simulink model "PB2M_001_003_RL"  (R2024a)
settings: Solver=FixedStepDiscrete  StartTime=0.0  StopTime=inf  FixedStep=[global_ST]  RelTol=1e-3
model workspace (MAT data in the model file):
  Var = 0
  imit_action_noise_variance = 0.2
values from neighbouring files (symbols this model uses):
  CGO2_cap = 5000    [SimControl_v3_rl.m]
  global_ST = 1    [SimControl_v3_rl.m]    (also in SimControl_v4.m)
  global_time = [0:1:8784]'    [SimControl_v3_rl.m]    (also in SimControl_v4.m)
undefined symbols (not defined in the file or in its folder): AEL, AMB, ATR, Bttry, CGO2, CHP, COMPR_MIX_E_spec, COMPR_SG_E_spec, DiscIntNeverNeededParam, DIST, DRY, forecast, GASF, Grd, MES, NumEpisodes, NumImitLearning, PV, th, vanilla, WT
libraries: simulink x1, slpidlib x1, rllib x1
(part 1 of 2)
settings Model: Creator=hogrebe  LastModifiedBy=salomon_p
settings SolverCC: AlgebraicLoopSolver=TrustRegion
settings DataIOCC: SaveState=on
settings OptimizationCC: BlockReduction=off
settings DebuggingCC: SignalInfNanChecking=error  UnconnectedInputMsg=warning  UnconnectedOutputMsg=warning  UnconnectedLineMsg=warning
settings ModelReferenceCC: EnableRefExpFcnMdlSchedulingChecks=on
settings RTWCC: GPUComputeCapability=3.5  DLArmComputeVersion=19.05

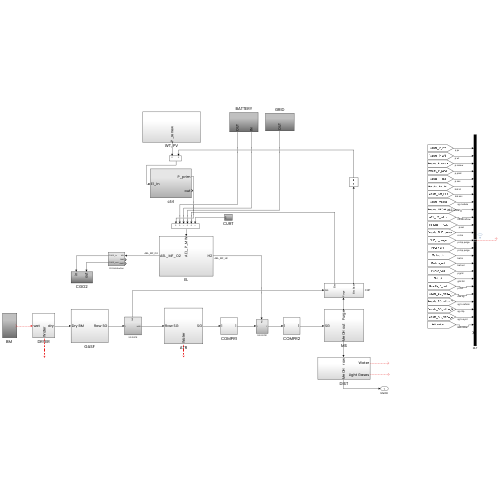
[thumbnail: Simulink's stored preview of the top-level diagram]
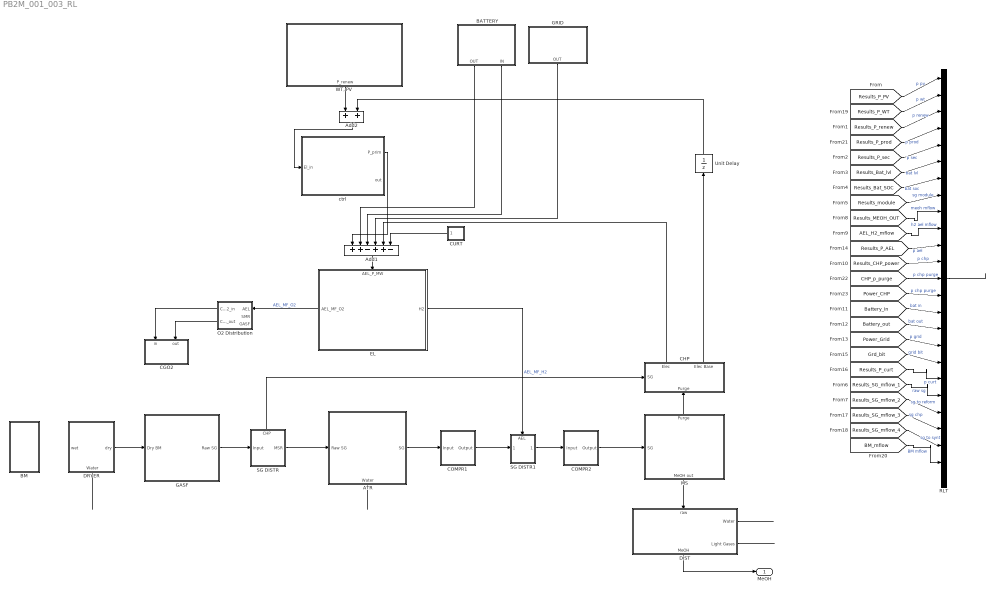
== system PB2M_001_003_RL ==
  ATR : Subsystem
      settings: PortSchema="{\"entries\":[{\"content\":{\"sides\":[{\"content\":{\"connectorIds\":[\"In1\"]},\"type\":\"ConnectorPlacement.EquallySpacedRectSide\",\"uuid\":\"d95d7370-a768-4e71-99c5-23d50f67aabe\"},{\"content\":{\"connectorIds\":[\"Out1\"],\"side\":\"RIGHT\"},\"type\":\"ConnectorPlacement.EquallySpacedRectSide\",\"uuid\":\"3437d418-ce7d-423d-8668-067a2caa5d39\"},{\"content\":{\"side\":\"TOP\"},\"type\":\"ConnectorPlacement.EquallySpacedRectSide\",\"uuid\":\"c8aa7c63-1393-4bbc-8660-d82006d9d42e\"},{\"content\":{\"connectorIds\":[\"Out2\"],\"side\":\"BOTTOM\"},\"type\":\"ConnectorPlacement.EquallySpacedRectSide\",\"uuid\":\"8d079498-92c7-4ac5-81b3-d100ec68b2bd\"}]},\"type\":\"ConnectorPlacement.EquallySpacedConnector\",\"uuid\":\"07712eec-a256-4c23-80e6-026550a38bce\"}],\"packageUris\":[\"http://schema.mathworks.com/mf0/Connector/R2020b\"],\"version\":\"1.0\"}"
  Add1 : Sum  Inputs=++-++-
  Add2 : Sum
  BATTERY : Subsystem
      settings: PortSchema="{\"entries\":[{\"content\":{\"sides\":[{\"content\":{},\"type\":\"ConnectorPlacement.EquallySpacedRectSide\",\"uuid\":\"b156ae25-26b3-4eee-ac7f-e302bdaac2ab\"},{\"content\":{\"side\":\"RIGHT\"},\"type\":\"ConnectorPlacement.EquallySpacedRectSide\",\"uuid\":\"f3a3b929-51c5-4419-b41e-ec6279a18565\"},{\"content\":{\"side\":\"TOP\"},\"type\":\"ConnectorPlacement.EquallySpacedRectSide\",\"uuid\":\"01f6443f-63f0-4718-804f-9bad3a04ddfb\"},{\"content\":{\"connectorIds\":[\"Out1\",\"Out2\"],\"side\":\"BOTTOM\"},\"type\":\"ConnectorPlacement.EquallySpacedRectSide\",\"uuid\":\"cbf48387-64e5-4e53-bde3-6e14dbb130f7\"}]},\"type\":\"ConnectorPlacement.EquallySpacedConnector\",\"uuid\":\"4aa34124-3e08-49a0-9db9-a8367ba9f9e9\"}],\"packageUris\":[\"http://schema.mathworks.com/mf0/Connector/R2020b\"],\"version\":\"1.0\"}"
  "BM " : Subsystem
  CGO2 : Subsystem
      settings: PortSchema="{\"entries\":[{\"content\":{\"sides\":[{\"content\":{},\"type\":\"ConnectorPlacement.EquallySpacedRectSide\",\"uuid\":\"5fd0e465-b758-40c5-99c0-bd502cf80220\"},{\"content\":{\"side\":\"RIGHT\"},\"type\":\"ConnectorPlacement.EquallySpacedRectSide\",\"uuid\":\"8c2bf71d-dd8a-4c38-9726-2100ecfb4157\"},{\"content\":{\"connectorIds\":[\"In1\",\"In2\"],\"side\":\"TOP\"},\"type\":\"ConnectorPlacement.EquallySpacedRectSide\",\"uuid\":\"9b00925e-eb9b-456e-968f-5d87047a8706\"}]},\"type\":\"ConnectorPlacement.EquallySpacedConnector\",\"uuid\":\"2f6cfec4-9fe2-41ff-9b0f-2d3a7383541d\"}],\"packageUris\":[\"http://schema.mathworks.com/mf0/Connector/R2020b\"],\"version\":\"1.0\"}"
  CHP : Subsystem
      settings: PortSchema="{\"entries\":[{\"content\":{\"sides\":[{\"content\":{\"connectorIds\":[\"In1\"]},\"type\":\"ConnectorPlacement.EquallySpacedRectSide\",\"uuid\":\"455e4cb2-b7ce-40b3-9267-45576cb92a35\"},{\"content\":{\"side\":\"RIGHT\"},\"type\":\"ConnectorPlacement.EquallySpacedRectSide\",\"uuid\":\"26266506-6e66-4bc0-bccd-a9e779dcae16\"},{\"content\":{\"connectorIds\":[\"Out1\",\"Out2\"],\"side\":\"TOP\"},\"type\":\"ConnectorPlacement.EquallySpacedRectSide\",\"uuid\":\"0bfe460e-97a8-4cdd-8918-1c56f22f3fbd\"},{\"content\":{\"connectorIds\":[\"In2\"],\"side\":\"BOTTOM\"},\"type\":\"ConnectorPlacement.EquallySpacedRectSide\",\"uuid\":\"d15a681e-1531-4d34-b913-d07bfab7e09a\"}]},\"type\":\"ConnectorPlacement.EquallySpacedConnector\",\"uuid\":\"864e4265-4fc9-4c94-8dd3-96a5c52575a2\"}],\"packageUris\":[\"http://schema.mathworks.com/mf0/Connector/R2020b\"],\"version\":\"1.0\"}"
  COMPR1 : Subsystem
  COMPR2 : Subsystem
  CURT : Subsystem
      settings: PortSchema="{\"entries\":[{\"content\":{\"sides\":[{\"content\":{\"connectorIds\":[\"Out1\"]},\"type\":\"ConnectorPlacement.EquallySpacedRectSide\",\"uuid\":\"455e4cb2-b7ce-40b3-9267-45576cb92a35\"},{\"content\":{\"side\":\"RIGHT\"},\"type\":\"ConnectorPlacement.EquallySpacedRectSide\",\"uuid\":\"26266506-6e66-4bc0-bccd-a9e779dcae16\"},{\"content\":{\"side\":\"TOP\"},\"type\":\"ConnectorPlacement.EquallySpacedRectSide\",\"uuid\":\"0bfe460e-97a8-4cdd-8918-1c56f22f3fbd\"}]},\"type\":\"ConnectorPlacement.EquallySpacedConnector\",\"uuid\":\"864e4265-4fc9-4c94-8dd3-96a5c52575a2\"}],\"packageUris\":[\"http://schema.mathworks.com/mf0/Connector/R2020b\"],\"version\":\"1.0\"}"
  DIST : Subsystem
      settings: PortSchema="{\"entries\":[{\"content\":{\"sides\":[{\"content\":{},\"type\":\"ConnectorPlacement.EquallySpacedRectSide\",\"uuid\":\"9bb20e76-c8c0-4ce3-bfa2-fd978c659bcc\"},{\"content\":{\"connectorIds\":[\"Out1\",\"Out2\"],\"side\":\"RIGHT\"},\"type\":\"ConnectorPlacement.EquallySpacedRectSide\",\"uuid\":\"12d31df4-77c9-4a5c-9a6c-fd7c89038c05\"},{\"content\":{\"connectorIds\":[\"In1\"],\"side\":\"TOP\"},\"type\":\"ConnectorPlacement.EquallySpacedRectSide\",\"uuid\":\"3a96496e-8d88-4b7f-91f0-6f8e8152b6d3\"},{\"content\":{\"connectorIds\":[\"Out3\"],\"side\":\"BOTTOM\"},\"type\":\"ConnectorPlacement.EquallySpacedRectSide\",\"uuid\":\"4bc833e2-fc0a-44a4-bcf0-3ebf0863e835\"}]},\"type\":\"ConnectorPlacement.EquallySpacedConnector\",\"uuid\":\"bb9c8f09-08c9-4a34-bdc9-5c844495fddc\"}],\"packageUris\":[\"http://schema.mathworks.com/mf0/Connector/R2020b\"],\"version\":\"1.0\"}"
  DRYER : Subsystem
      settings: PortSchema="{\"entries\":[{\"content\":{\"sides\":[{\"content\":{},\"type\":\"ConnectorPlacement.EquallySpacedRectSide\",\"uuid\":\"4ebfcccc-776f-4872-9d0b-9643b5960bad\"},{\"content\":{\"connectorIds\":[\"Out1\"],\"side\":\"RIGHT\"},\"type\":\"ConnectorPlacement.EquallySpacedRectSide\",\"uuid\":\"52af1a20-21ba-42da-ac0d-5cc3ed928415\"},{\"content\":{\"connectorIds\":[\"Out2\"],\"side\":\"TOP\"},\"type\":\"ConnectorPlacement.EquallySpacedRectSide\",\"uuid\":\"35b3f618-6f56-49d4-89a8-2314405479bc\"},{\"content\":{\"connectorIds\":[\"In1\"],\"side\":\"BOTTOM\"},\"type\":\"ConnectorPlacement.EquallySpacedRectSide\",\"uuid\":\"a7ad5d18-a31c-4405-a5bd-3fe59bb19813\"}]},\"type\":\"ConnectorPlacement.EquallySpacedConnector\",\"uuid\":\"90f717a7-269d-4abb-8032-a33661c35212\"}],\"packageUris\":[\"http://schema.mathworks.com/mf0/Connector/R2020b\"],\"version\":\"1.0\"}"
  EL : Subsystem
      settings: PortSchema="{\"entries\":[{\"content\":{\"sides\":[{\"content\":{\"connectorIds\":[\"Out2\"]},\"type\":\"ConnectorPlacement.EquallySpacedRectSide\",\"uuid\":\"e86b81d9-d45f-45ad-8c80-2ef5c9159145\"},{\"content\":{\"connectorIds\":[\"Out1\"],\"side\":\"RIGHT\"},\"type\":\"ConnectorPlacement.EquallySpacedRectSide\",\"uuid\":\"b091bd34-fe91-455d-8135-92fc1e1b5bd7\"},{\"content\":{\"connectorIds\":[\"In1\"],\"side\":\"TOP\"},\"type\":\"ConnectorPlacement.EquallySpacedRectSide\",\"uuid\":\"804c6318-ad33-4a07-b17e-e0d2fd6b4b2f\"}]},\"type\":\"ConnectorPlacement.EquallySpacedConnector\",\"uuid\":\"e581105a-7c66-468d-8489-1abddd5a4bb6\"}],\"packageUris\":[\"http://schema.mathworks.com/mf0/Connector/R2020b\"],\"version\":\"1.0\"}"
  GASF : Subsystem
  GRID : Subsystem
      settings: PortSchema="{\"entries\":[{\"content\":{\"sides\":[{\"content\":{},\"type\":\"ConnectorPlacement.EquallySpacedRectSide\",\"uuid\":\"13ddf689-c473-4fae-8488-05ba2c53be01\"},{\"content\":{\"side\":\"RIGHT\"},\"type\":\"ConnectorPlacement.EquallySpacedRectSide\",\"uuid\":\"3edd6540-09f8-47a0-8af0-925a1a207bbe\"},{\"content\":{\"side\":\"TOP\"},\"type\":\"ConnectorPlacement.EquallySpacedRectSide\",\"uuid\":\"e7e0af70-0c4e-4701-890f-2bc2f1b60263\"},{\"content\":{\"connectorIds\":[\"Out1\"],\"side\":\"BOTTOM\"},\"type\":\"ConnectorPlacement.EquallySpacedRectSide\",\"uuid\":\"aae9c7fc-ae1b-458f-888e-dcbddd5e368f\"}]},\"type\":\"ConnectorPlacement.EquallySpacedConnector\",\"uuid\":\"9fa59c12-9be8-49ba-a862-8cdac5f592f4\"}],\"packageUris\":[\"http://schema.mathworks.com/mf0/Connector/R2020b\"],\"version\":\"1.0\"}"
  MS : Subsystem
      settings: PortSchema="{\"entries\":[{\"content\":{\"sides\":[{\"content\":{\"connectorIds\":[\"In1\"]},\"type\":\"ConnectorPlacement.EquallySpacedRectSide\",\"uuid\":\"7c68cb95-e770-413e-a40e-672fd8604812\"},{\"content\":{\"side\":\"RIGHT\"},\"type\":\"ConnectorPlacement.EquallySpacedRectSide\",\"uuid\":\"6240a65a-2dbc-4a6e-817e-2ab31946396e\"},{\"content\":{\"connectorIds\":[\"Out2\"],\"side\":\"TOP\"},\"type\":\"ConnectorPlacement.EquallySpacedRectSide\",\"uuid\":\"1a1b519e-0693-45b9-a906-950b0dca57a1\"},{\"content\":{\"connectorIds\":[\"Out1\"],\"side\":\"BOTTOM\"},\"type\":\"ConnectorPlacement.EquallySpacedRectSide\",\"uuid\":\"e87dd805-e630-4a2f-8388-2c51cd14fe9e\"}]},\"type\":\"ConnectorPlacement.EquallySpacedConnector\",\"uuid\":\"e16e5d91-de04-48fc-b44b-fdb042a92f84\"}],\"packageUris\":[\"http://schema.mathworks.com/mf0/Connector/R2020b\"],\"version\":\"1.0\"}"
  O2 Distribution : Subsystem
      settings: PortSchema="{\"entries\":[{\"content\":{\"sides\":[{\"content\":{\"connectorIds\":[\"Out3\",\"Out4\"]},\"type\":\"ConnectorPlacement.EquallySpacedRectSide\",\"uuid\":\"30156f9c-db5e-4257-aeed-83f2c1c2e5bf\"},{\"content\":{\"connectorIds\":[\"In1\",\"Out1\",\"Out2\"],\"side\":\"RIGHT\"},\"type\":\"ConnectorPlacement.EquallySpacedRectSide\",\"uuid\":\"c3a4c4df-5b27-475f-87a9-b45da9a3b436\"},{\"content\":{\"side\":\"TOP\"},\"type\":\"ConnectorPlacement.EquallySpacedRectSide\",\"uuid\":\"5997053d-e240-46ef-b6d7-4f9a3a1c0d15\"}]},\"type\":\"ConnectorPlacement.EquallySpacedConnector\",\"uuid\":\"10d495fb-251b-444d-bd0a-f6bbcb16daf1\"}],\"packageUris\":[\"http://schema.mathworks.com/mf0/Connector/R2020b\"],\"version\":\"1.0\"}"
  RLT : BusCreator  Inputs=25
  SG DISTR : Subsystem
      settings: PortSchema="{\"entries\":[{\"content\":{\"sides\":[{\"content\":{},\"type\":\"ConnectorPlacement.EquallySpacedRectSide\",\"uuid\":\"e86b81d9-d45f-45ad-8c80-2ef5c9159145\"},{\"content\":{\"connectorIds\":[\"Out1\"],\"side\":\"RIGHT\"},\"type\":\"ConnectorPlacement.EquallySpacedRectSide\",\"uuid\":\"b091bd34-fe91-455d-8135-92fc1e1b5bd7\"},{\"content\":{\"connectorIds\":[\"In1\"],\"side\":\"TOP\"},\"type\":\"ConnectorPlacement.EquallySpacedRectSide\",\"uuid\":\"804c6318-ad33-4a07-b17e-e0d2fd6b4b2f\"},{\"content\":{\"connectorIds\":[\"Out2\"],\"side\":\"BOTTOM\"},\"type\":\"ConnectorPlacement.EquallySpacedRectSide\",\"uuid\":\"fb2b571c-70ad-41c0-9018-552f5e98e285\"}]},\"type\":\"ConnectorPlacement.EquallySpacedConnector\",\"uuid\":\"e581105a-7c66-468d-8489-1abddd5a4bb6\"}],\"packageUris\":[\"http://schema.mathworks.com/mf0/Connector/R2020b\"],\"version\":\"1.0\"}"
  SG DISTR1 : Subsystem
      settings: PortSchema="{\"entries\":[{\"content\":{\"sides\":[{\"content\":{},\"type\":\"ConnectorPlacement.EquallySpacedRectSide\",\"uuid\":\"e9c91cab-8c69-4152-b789-7325d2e32e4b\"},{\"content\":{\"connectorIds\":[\"In2\"],\"side\":\"RIGHT\"},\"type\":\"ConnectorPlacement.EquallySpacedRectSide\",\"uuid\":\"b801369b-5c93-4438-bd90-0992b326086c\"},{\"content\":{\"connectorIds\":[\"In1\"],\"side\":\"TOP\"},\"type\":\"ConnectorPlacement.EquallySpacedRectSide\",\"uuid\":\"e103e961-9a42-4e45-906c-e9068e5e276c\"},{\"content\":{\"connectorIds\":[\"Out1\"],\"side\":\"BOTTOM\"},\"type\":\"ConnectorPlacement.EquallySpacedRectSide\",\"uuid\":\"0e96afff-5922-401c-b36e-06eb0842909a\"}]},\"type\":\"ConnectorPlacement.EquallySpacedConnector\",\"uuid\":\"2ea93f77-6b27-4245-9c93-a72fb1fe7fa6\"}],\"packageUris\":[\"http://schema.mathworks.com/mf0/Connector/R2020b\"],\"version\":\"1.0\"}"
  Unit Delay : UnitDelay  SampleTime=-1  HasFrameUpgradeWarning=on
  "WT, PV" : Subsystem
      settings: PortSchema="{\"entries\":[{\"content\":{\"sides\":[{\"content\":{},\"type\":\"ConnectorPlacement.EquallySpacedRectSide\",\"uuid\":\"8a2d1ae0-dccb-4b14-8547-5eeedb1731af\"},{\"content\":{\"side\":\"RIGHT\"},\"type\":\"ConnectorPlacement.EquallySpacedRectSide\",\"uuid\":\"3fb157a2-f839-4f36-8a45-db822d022818\"},{\"content\":{\"side\":\"TOP\"},\"type\":\"ConnectorPlacement.EquallySpacedRectSide\",\"uuid\":\"528eda02-61b1-46fc-814d-d4347d4497c7\"},{\"content\":{\"connectorIds\":[\"Out1\"],\"side\":\"BOTTOM\"},\"type\":\"ConnectorPlacement.EquallySpacedRectSide\",\"uuid\":\"9515b46c-adb3-49ca-b783-afbfd8bcb61a\"}]},\"type\":\"ConnectorPlacement.EquallySpacedConnector\",\"uuid\":\"11973188-1db2-4f1c-be62-25a3f427210a\"}],\"packageUris\":[\"http://schema.mathworks.com/mf0/Connector/R2020b\"],\"version\":\"1.0\"}"
  ctrl : Subsystem
  MeOH : Outport
  wires:
  EL/2(AEL_MF_O2) -> O2 Distribution/1(AEL)  "AEL_MF_O2"
  O2 Distribution/4(CGO2_out) -> CGO2/2(out)
  O2 Distribution/3(CGO2_in) -> CGO2/1(in)
  SG DISTR/2(MSR) -> ATR/1(Raw SG)
  DRYER/2(dry) -> GASF/1(Dry BM)
  GASF/1(Raw SG) -> SG DISTR/1(Input)
  EL/1(H2) -> SG DISTR1/2(AEL)  "AEL_MF_H2"
  ATR/1(SG) -> COMPR1/1(Input)
  SG DISTR1/1(Output) -> COMPR2/1(Input)
  SG DISTR/1(CHP) -> CHP/1(SG)
  ? -> DRYER/1(wet)
  COMPR2/1(Output) -> MS/1(SG)
  ctrl/1(P_prim) -> Add1/1
  Add1/1 -> EL/1(AEL_P_MW)
  CHP/1(Elec) -> Add1/5
  BATTERY/1(OUT) -> Add1/2
  BATTERY/2(IN) -> Add1/3
  GRID/1(OUT) -> Add1/4
  CURT/1(Output) -> Add1/6
  COMPR1/1(Output) -> SG DISTR1/1(Input1)
  RLT/1 -> ?
  [Results_SG_mflow_4] -> RLT/23  "sg to synt"
  [Results_SG_mflow_2] -> RLT/21  "sg to reform"
  [Results_P_curt] -> RLT/19  "p curt"
  [Results_P_PV] -> RLT/1  "p pv"
  [Grd_bit] -> RLT/18  "grid bit"
  [Results_P_renew] -> RLT/3  "p renew"
  [Power_Grid] -> RLT/17  "p grid"
  [Results_CHP_power] -> RLT/12  "p chp"
  [Battery_out] -> RLT/16  "bat out"
  [Results_module] -> RLT/8  "sg module"
  [Battery_in] -> RLT/15  "bat in"
  [Results_P_AEL] -> RLT/11  "p ael"
  [AEL_H2_mflow] -> RLT/10  "h2 ael mflow"
  [Results_Bat_SOC] -> RLT/7  "bat soc"
  [Results_Bat_lvl] -> RLT/6  "bat lvl"
  [Results_MEOH_OUT] -> RLT/9  "meoh mflow"
  [Results_SG_mflow_1] -> RLT/20  "raw sg"
  [Results_P_sec] -> RLT/5  "p sec"
  [Results_SG_mflow_3] -> RLT/22  "sg chp"
  MS/2(Purge) -> CHP/2(Purge)
  Add2/1 -> ctrl/1(El_in)
  "WT, PV"/1(P_renew) -> Add2/1
  CHP/2(Elec Base) -> Unit Delay/1
  DRYER/1(Water) -> ?
  ATR/2(Water) -> ?
  MS/1(MeOH out) -> DIST/1(raw)
  DIST/3(MeOH) -> MeOH/1
  DIST/1(Water) -> ?
  DIST/2(Light Gases) -> ?
  [BM_mflow] -> RLT/24  "BM mflow"
  [Results_P_prod] -> RLT/4  "p prod"
  [CHP_p_purge] -> RLT/13  "p chp purge"
  [Power_CHP] -> RLT/14  "p chp purge"
  [Results_P_WT] -> RLT/2  "p wt"
  Unit Delay/1 -> Add2/2

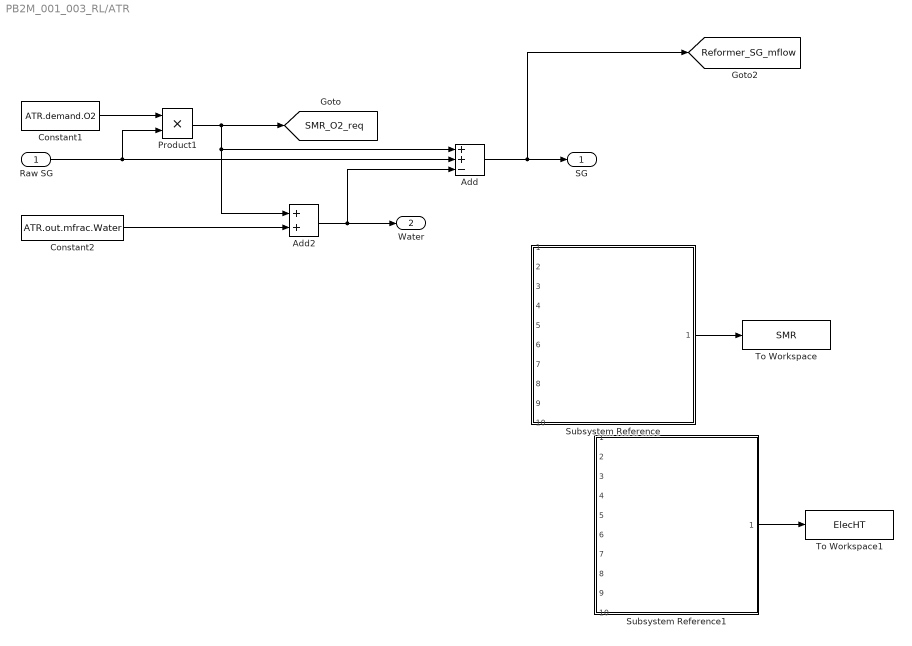
== system PB2M_001_003_RL/ATR ==
  Raw SG : Inport
  Add : Sum  Inputs=++-
  Add2 : Sum
  Constant1 : Constant  Value=ATR.demand.O2
  Constant2 : Constant  Value=ATR.out.mfrac.Water
  Product1 : Product
  Subsystem Reference : Subsystem  ReferencedSubsystem=Output_generation
  Subsystem Reference1 : Subsystem  ReferencedSubsystem=Output_generation
  To Workspace : ToWorkspace  VariableName=SMR  SampleTime=-1
  To Workspace1 : ToWorkspace  VariableName=ElecHT  SampleTime=-1
  SG : Outport
  Water : Outport  Port=2
  tag scope: Reformer_SG_mflow=global, SMR_O2_req=global
  wires:
  Subsystem Reference/1 -> To Workspace/1
  Constant1/1 -> Product1/1
  Product1/1 -> Add/1, Add2/1, [SMR_O2_req]
  Raw SG/1 -> Add/2, Product1/2
  Constant2/1 -> Add2/2
  Add2/1 -> Add/3, Water/1
  Add/1 -> [Reformer_SG_mflow], SG/1
  Subsystem Reference1/1 -> To Workspace1/1

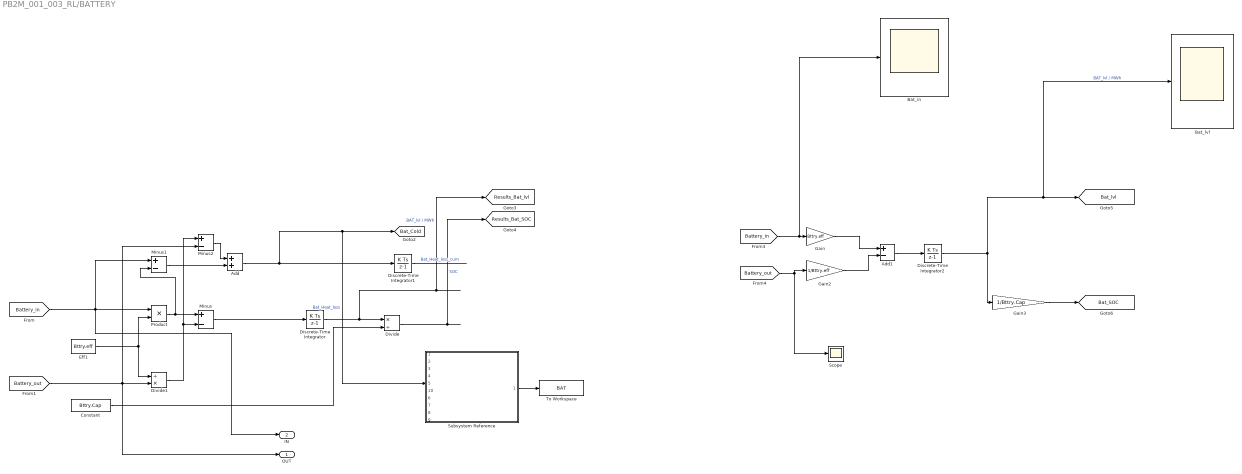
== system PB2M_001_003_RL/BATTERY ==
  Add : Sum
  Add1 : Sum  Inputs=+-
  Bat_in : Scope
  Bat_lvl : Scope
  Constant : Constant  Value=Bttry.Cap
  Discrete-Time Integrator : DiscreteIntegrator  SampleTime=-1  ICPrevOutput=DiscIntNeverNeededParam  ICPrevScaledInput=DiscIntNeverNeededParam
  Discrete-Time Integrator1 : DiscreteIntegrator  SampleTime=-1  ICPrevOutput=DiscIntNeverNeededParam  ICPrevScaledInput=DiscIntNeverNeededParam
  Discrete-Time Integrator2 : DiscreteIntegrator  InitialCondition=Bttry.min  SampleTime=-1  LimitOutput=on  UpperSaturationLimit=Bttry.Cap  LowerSaturationLimit=Bttry.min  ICPrevOutput=DiscIntNeverNeededParam  ICPrevScaledInput=DiscIntNeverNeededParam
  Divide : Product  Inputs=*/
  Divide1 : Product  Inputs=/*
  Eff1 : Constant  Value=Bttry.eff
  Gain : Gain  Gain=Bttry.eff
  Gain2 : Gain  Gain=1/Bttry.eff
  Gain3 : Gain  Gain=1/Bttry.Cap
  Minus : Sum  Inputs=+-
  Minus1 : Sum  Inputs=+-
  Minus2 : Sum  Inputs=+-
  Product : Product
  Scope : Scope
  Subsystem Reference : Subsystem  ReferencedSubsystem=Output_generation
      settings: PortSchema="{\"entries\":[{\"content\":{\"sides\":[{\"content\":{\"connectorIds\":[\"In1\",\"In2\",\"In3\",\"In4\",\"In5\",\"In10\",\"In6\",\"In7\",\"In8\",\"In9\"]},\"type\":\"ConnectorPlacement.EquallySpacedRectSide\",\"uuid\":\"21c211f6-d300-429e-920b-eada30affdb6\"},{\"content\":{\"connectorIds\":[\"Out1\"],\"side\":\"RIGHT\"},\"type\":\"ConnectorPlacement.EquallySpacedRectSide\",\"uuid\":\"b1fcdfee-52f7-4682-8799-22b33d08abbf\"},{\"content\":{\"side\":\"TOP\"},\"type\":\"ConnectorPlacement.EquallySpacedRectSide\",\"uuid\":\"5cecd853-e592-48b7-a1a6-516483ee8138\"}]},\"type\":\"ConnectorPlacement.EquallySpacedConnector\",\"uuid\":\"0d6337ce-2718-4de2-80e8-a88f22d313ea\"}],\"packageUris\":[\"http://schema.mathworks.com/mf0/Connector/R2020b\"],\"version\":\"1.0\"}"
  To Workspace : ToWorkspace  VariableName=BAT  SampleTime=-1
  OUT : Outport
  IN : Outport  Port=2
  tag scope: Bat_Cold=global, Bat_SOC=global, Bat_lvl=global, Results_Bat_SOC=global, Results_Bat_lvl=global
  wires:
  Constant/1 -> Divide/2
  Divide/1 -> [Results_Bat_SOC]  "SOC"
  Product/1 -> Minus1/2, Minus/1
  Divide1/1 -> Minus2/1, Minus/2
  Eff1/1 -> Divide1/1, Product/2
  Discrete-Time Integrator/1 -> [Results_Bat_lvl], Divide/1  "BAT_lvl / MWh"
  Subsystem Reference/1 -> To Workspace/1
  Minus1/1 -> Add/2
  Minus2/1 -> Add/1
  Add/1 -> [Bat_Cold], Subsystem Reference/5, Discrete-Time Integrator1/1  "Bat_Heat_loss"
  Discrete-Time Integrator1/1 -> ?  "Bat_Heat_loss_cum"
  [Battery_out] -> Divide1/2, OUT/1, Minus2/2
  [Battery_in] -> IN/1, Minus1/1, Product/1
  Minus/1 -> Discrete-Time Integrator/1
  [Battery_in] -> Bat_in/1, Gain/1
  [Battery_out] -> Scope/1, Gain2/1
  Gain2/1 -> Add1/2
  Add1/1 -> Discrete-Time Integrator2/1
  Gain/1 -> Add1/1
  Discrete-Time Integrator2/1 -> Bat_lvl/1, [Bat_lvl], Gain3/1  "BAT_lvl / MWh"
  Gain3/1 -> [Bat_SOC]

== system PB2M_001_003_RL/BM  ==
  IC : InitialCondition
  MATLAB Function : MATLAB Function  TreatAsAtomicUnit=on
  Unit Delay : UnitDelay  SampleTime=-1  HasFrameUpgradeWarning=on
  Unit Delay1 : UnitDelay  SampleTime=-1  HasFrameUpgradeWarning=on
  tag scope: Results_module=global
  wires:
  [AEL_H2_mflow] -> Unit Delay/1
  [Reformer_SG_mflow] -> Unit Delay1/1
  MATLAB Function/1(module) -> IC/1
  IC/1 -> [Results_module]
  Unit Delay/1 -> MATLAB Function/1(mflow_H2)
  Unit Delay1/1 -> MATLAB Function/2(mflow_SG)

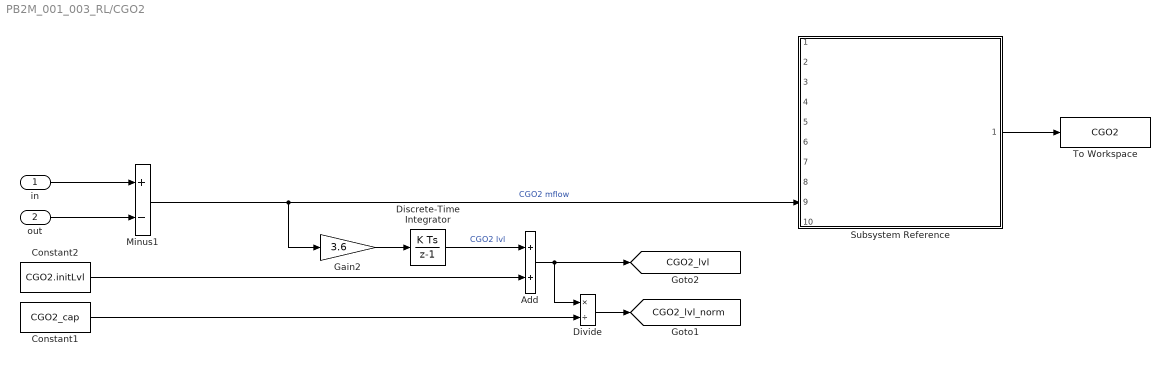
== system PB2M_001_003_RL/CGO2 ==
  in : Inport
  out : Inport  Port=2
  Add : Sum
  Constant1 : Constant  Value=CGO2_cap
  Constant2 : Constant  Value=CGO2.initLvl
  Discrete-Time Integrator : DiscreteIntegrator  SampleTime=-1  ICPrevOutput=DiscIntNeverNeededParam  ICPrevScaledInput=DiscIntNeverNeededParam
  Divide : Product  Inputs=*/
  Gain2 : Gain  Gain=3.6
  Minus1 : Sum  Inputs=+-
  Subsystem Reference : Subsystem  ReferencedSubsystem=Output_generation
  To Workspace : ToWorkspace  VariableName=CGO2  SampleTime=-1
  tag scope: CGO2_lvl=global, CGO2_lvl_norm=global
  wires:
  in/1 -> Minus1/1
  out/1 -> Minus1/2
  Minus1/1 -> Gain2/1, Subsystem Reference/9  "CGO2 mflow"
  Subsystem Reference/1 -> To Workspace/1
  Gain2/1 -> Discrete-Time Integrator/1
  Discrete-Time Integrator/1 -> Add/1  "CGO2 lvl"
  Constant2/1 -> Add/2
  Add/1 -> Divide/1, [CGO2_lvl]
  Constant1/1 -> Divide/2
  Divide/1 -> [CGO2_lvl_norm]

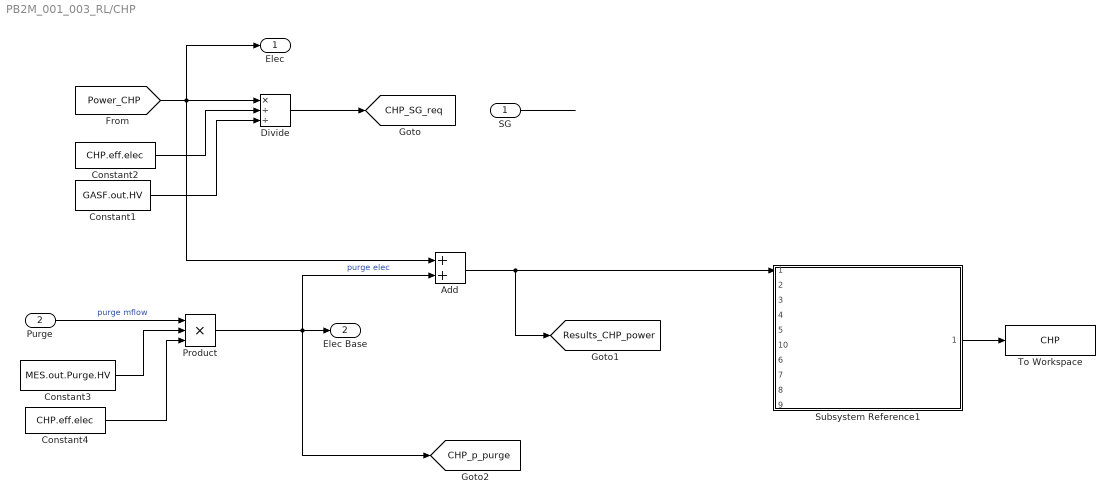
== system PB2M_001_003_RL/CHP ==
  SG : Inport
  Purge : Inport  Port=2
  Add : Sum
  Constant1 : Constant  Value=GASF.out.HV
  Constant2 : Constant  Value=CHP.eff.elec
  Constant3 : Constant  Value=MES.out.Purge.HV
  Constant4 : Constant  Value=CHP.eff.elec
  Divide : Product  Inputs=*//
  Product : Product  Inputs=***
  Subsystem Reference1 : Subsystem  ReferencedSubsystem=Output_generation
      settings: PortSchema="{\"entries\":[{\"content\":{\"sides\":[{\"content\":{\"connectorIds\":[\"In1\",\"In2\",\"In3\",\"In4\",\"In5\",\"In10\",\"In6\",\"In7\",\"In8\",\"In9\"]},\"type\":\"ConnectorPlacement.EquallySpacedRectSide\",\"uuid\":\"21c211f6-d300-429e-920b-eada30affdb6\"},{\"content\":{\"connectorIds\":[\"Out1\"],\"side\":\"RIGHT\"},\"type\":\"ConnectorPlacement.EquallySpacedRectSide\",\"uuid\":\"b1fcdfee-52f7-4682-8799-22b33d08abbf\"},{\"content\":{\"side\":\"TOP\"},\"type\":\"ConnectorPlacement.EquallySpacedRectSide\",\"uuid\":\"5cecd853-e592-48b7-a1a6-516483ee8138\"}]},\"type\":\"ConnectorPlacement.EquallySpacedConnector\",\"uuid\":\"0d6337ce-2718-4de2-80e8-a88f22d313ea\"}],\"packageUris\":[\"http://schema.mathworks.com/mf0/Connector/R2020b\"],\"version\":\"1.0\"}"
  To Workspace : ToWorkspace  VariableName=CHP  SampleTime=-1
  Elec : Outport
  Elec Base : Outport  Port=2
  tag scope: CHP_SG_req=global, CHP_p_purge=global, Results_CHP_power=global
  wires:
  Divide/1 -> [CHP_SG_req]
  [Power_CHP] -> Add/1, Elec/1, Divide/1
  Constant2/1 -> Divide/2
  Constant1/1 -> Divide/3
  Subsystem Reference1/1 -> To Workspace/1
  Purge/1 -> Product/1  "purge mflow"
  Constant3/1 -> Product/2
  Constant4/1 -> Product/3
  Product/1 -> [CHP_p_purge], Elec Base/1, Add/2  "purge elec"
  Add/1 -> [Results_CHP_power], Subsystem Reference1/1
  SG/1 -> ?

== system PB2M_001_003_RL/COMPR1 ==
  Input : Inport
  Constant : Constant  Value=COMPR_SG_E_spec
  Product : Product
  Output : Outport
  tag scope: COMPR_1_E=global
  wires:
  Constant/1 -> Product/1
  Input/1 -> Product/2
  Product/1 -> Output/1, [COMPR_1_E]

== system PB2M_001_003_RL/COMPR2 ==
  Input : Inport
  Constant : Constant  Value=COMPR_MIX_E_spec
  Product : Product
  Output : Outport
  tag scope: COMPR_2_E=global
  wires:
  Constant/1 -> Product/1
  Input/1 -> Product/2
  Product/1 -> Output/1, [COMPR_2_E]

== system PB2M_001_003_RL/CURT ==
  Output : Outport
  wires:
  [Results_P_curt] -> Output/1

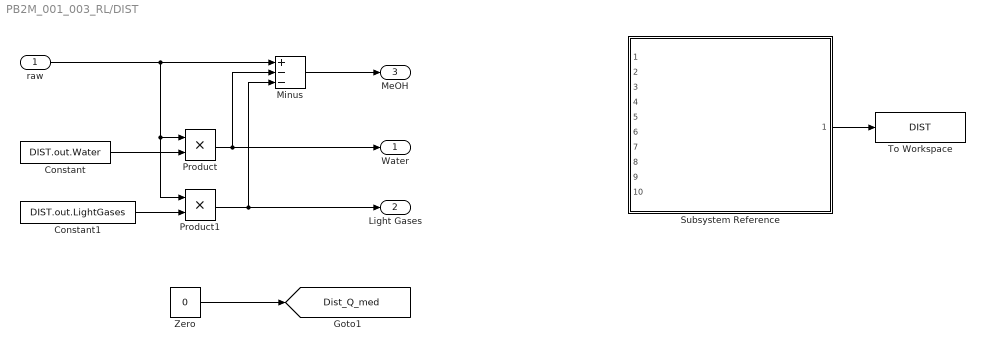
== system PB2M_001_003_RL/DIST ==
  raw : Inport
  Constant : Constant  Value=DIST.out.Water
  Constant1 : Constant  Value=DIST.out.LightGases
  Minus : Sum  Inputs=+--
  Product : Product
  Product1 : Product
  Subsystem Reference : Subsystem  ReferencedSubsystem=Output_generation
  To Workspace : ToWorkspace  VariableName=DIST  SampleTime=-1
  Zero : Constant  Value=0  OutDataTypeStr=Inherit: Inherit via back propagation
  Water : Outport
  Light Gases : Outport  Port=2
  MeOH : Outport  Port=3
  tag scope: Dist_Q_med=global
  wires:
  Subsystem Reference/1 -> To Workspace/1
  Zero/1 -> [Dist_Q_med]
  raw/1 -> Minus/1, Product1/1, Product/1
  Constant/1 -> Product/2
  Product/1 -> Water/1, Minus/2
  Constant1/1 -> Product1/2
  Product1/1 -> Light Gases/1, Minus/3
  Minus/1 -> MeOH/1

== system PB2M_001_003_RL/DRYER ==
  wet : Inport
  Constant1 : Constant  Value=DRY.demand.P
  Constant2 : Constant  Value=DRY.out.H2O.mflow
  Minus : Sum  Inputs=+-
  Product : Product
  Product3 : Product
  Subsystem Reference1 : Subsystem  ReferencedSubsystem=Output_generation
      settings: PortSchema="{\"entries\":[{\"content\":{\"sides\":[{\"content\":{\"connectorIds\":[\"In1\",\"In2\",\"In3\",\"In4\",\"In5\",\"In10\",\"In6\",\"In7\",\"In8\",\"In9\"]},\"type\":\"ConnectorPlacement.EquallySpacedRectSide\",\"uuid\":\"21c211f6-d300-429e-920b-eada30affdb6\"},{\"content\":{\"connectorIds\":[\"Out1\"],\"side\":\"RIGHT\"},\"type\":\"ConnectorPlacement.EquallySpacedRectSide\",\"uuid\":\"b1fcdfee-52f7-4682-8799-22b33d08abbf\"},{\"content\":{\"side\":\"TOP\"},\"type\":\"ConnectorPlacement.EquallySpacedRectSide\",\"uuid\":\"5cecd853-e592-48b7-a1a6-516483ee8138\"}]},\"type\":\"ConnectorPlacement.EquallySpacedConnector\",\"uuid\":\"0d6337ce-2718-4de2-80e8-a88f22d313ea\"}],\"packageUris\":[\"http://schema.mathworks.com/mf0/Connector/R2020b\"],\"version\":\"1.0\"}"
  To Workspace1 : ToWorkspace  VariableName=DRYER  SampleTime=-1
  Water : Outport
  dry : Outport  Port=2
  tag scope: DRY_E=global
  wires:
  wet/1 -> Minus/1, Product/1
  Subsystem Reference1/1 -> To Workspace1/1
  Minus/1 -> dry/1, Product3/1
  Product/1 -> Minus/2, Water/1
  Constant1/1 -> Product3/2
  Product3/1 -> [DRY_E]
  Constant2/1 -> Product/2

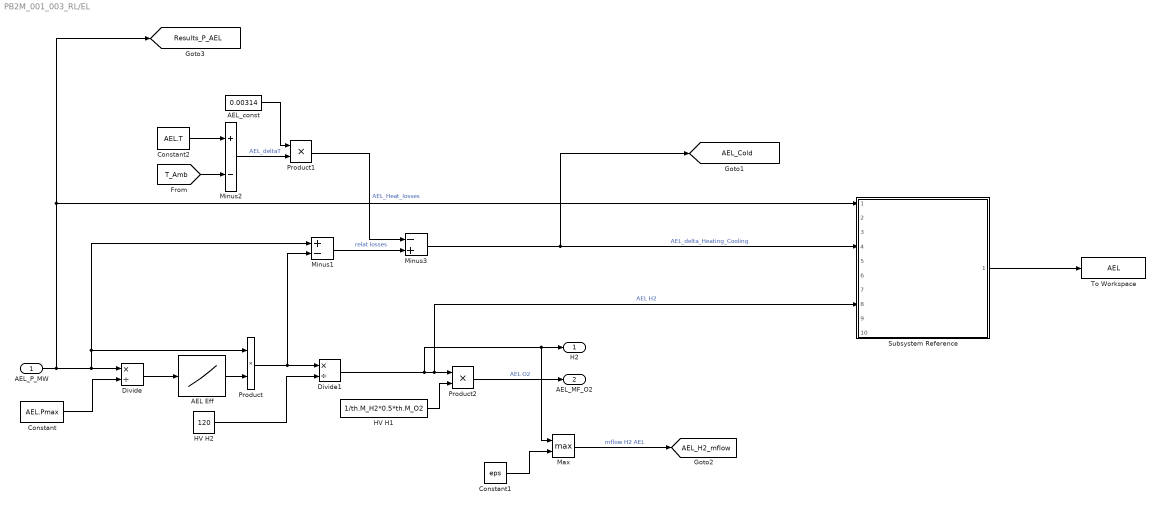
== system PB2M_001_003_RL/EL ==
  AEL_P_MW : Inport
  AEL Eff : Lookup_n-D  NumberOfTableDimensions=1  BreakpointsForDimension1=[AEL.LU.relatPower]'  Table=[AEL.LU.Eff]'  InternalRulePriority=Speed  RndMeth=Simplest
  AEL_const : Constant  Value=0.00314
  Constant : Constant  Value=AEL.Pmax
  Constant1 : Constant  Value=eps
  Constant2 : Constant  Value=AEL.T
  Divide : Product  Inputs=*/
  Divide1 : Product  Inputs=*/
  HV H1 : Constant  Value=1/th.M_H2*0.5*th.M_O2
  HV H2 : Constant  Value=120
  Max : MinMax  Function=max  Inputs=2
  Minus1 : Sum  Inputs=+-
  Minus2 : Sum  Inputs=+-
  Minus3 : Sum  Inputs=-+
  Product : Product
  Product1 : Product
  Product2 : Product
  Subsystem Reference : Subsystem  ReferencedSubsystem=Output_generation
  To Workspace : ToWorkspace  VariableName=AEL  SampleTime=-1
  H2 : Outport
  AEL_MF_O2 : Outport  Port=2
  tag scope: AEL_Cold=global, AEL_H2_mflow=global, Results_P_AEL=global
  wires:
  Divide/1 -> AEL Eff/1
  Product2/1 -> AEL_MF_O2/1  "AEL O2"
  Subsystem Reference/1 -> To Workspace/1
  AEL Eff/1 -> Product/2
  Product/1 -> Divide1/1, Minus1/2
  HV H2/1 -> Divide1/2
  AEL_P_MW/1 -> [Results_P_AEL], Subsystem Reference/1, Divide/1, Product/1, Minus1/1
  Minus1/1 -> Minus3/2  "relat losses"
  Constant2/1 -> Minus2/1
  [T_Amb] -> Minus2/2
  Minus2/1 -> Product1/2  "AEL_deltaT"
  Minus3/1 -> [AEL_Cold], Subsystem Reference/4  "AEL_delta_Heating_Cooling"
  AEL_const/1 -> Product1/1
  Product1/1 -> Minus3/1  "AEL_Heat_losses"
  Divide1/1 -> Max/1, H2/1, Subsystem Reference/8, Product2/1  "AEL H2"
  HV H1/1 -> Product2/2
  Constant1/1 -> Max/2
  Max/1 -> [AEL_H2_mflow]  "mflow H2 AEL"
  Constant/1 -> Divide/2

== system PB2M_001_003_RL/GASF ==
  Dry BM : Inport
  Add : Sum  Inputs=3
  Constant : Constant  Value=GASF.demand.O2
  Constant1 : Constant  Value=GASF.demand.Steam
  Product : Product
  Product1 : Product
  Subsystem Reference1 : Subsystem  ReferencedSubsystem=Output_generation
      settings: PortSchema="{\"entries\":[{\"content\":{\"sides\":[{\"content\":{\"connectorIds\":[\"In1\",\"In2\",\"In3\",\"In4\",\"In5\",\"In10\",\"In6\",\"In7\",\"In8\",\"In9\"]},\"type\":\"ConnectorPlacement.EquallySpacedRectSide\",\"uuid\":\"21c211f6-d300-429e-920b-eada30affdb6\"},{\"content\":{\"connectorIds\":[\"Out1\"],\"side\":\"RIGHT\"},\"type\":\"ConnectorPlacement.EquallySpacedRectSide\",\"uuid\":\"b1fcdfee-52f7-4682-8799-22b33d08abbf\"},{\"content\":{\"side\":\"TOP\"},\"type\":\"ConnectorPlacement.EquallySpacedRectSide\",\"uuid\":\"5cecd853-e592-48b7-a1a6-516483ee8138\"}]},\"type\":\"ConnectorPlacement.EquallySpacedConnector\",\"uuid\":\"0d6337ce-2718-4de2-80e8-a88f22d313ea\"}],\"packageUris\":[\"http://schema.mathworks.com/mf0/Connector/R2020b\"],\"version\":\"1.0\"}"
  To Workspace1 : ToWorkspace  VariableName=GASF  SampleTime=-1
  Raw SG : Outport
  tag scope: GASF_O2_req=global, GASF_STEAM_req=global, Results_SG_mflow_1=global
  wires:
  Constant/1 -> Product/1
  Dry BM/1 -> Product1/2, Product/2, Add/3
  Constant1/1 -> Product1/1
  Product1/1 -> Add/1, [GASF_STEAM_req]
  Product/1 -> Add/2, [GASF_O2_req]
  Add/1 -> [Results_SG_mflow_1], Raw SG/1
  Subsystem Reference1/1 -> To Workspace1/1

== system PB2M_001_003_RL/GRID ==
  Digital Clock : DigitalClock  SampleTime=[global_ST]
  MATLAB Function : MATLAB Function  TreatAsAtomicUnit=on
  MATLAB Function1 : MATLAB Function  TreatAsAtomicUnit=on
  Subsystem Reference : Subsystem  ReferencedSubsystem=Output_generation
  To Workspace : ToWorkspace  VariableName=Grid  SampleTime=-1
  daily_Grid_costs : Lookup_n-D  NumberOfTableDimensions=1  BreakpointsForDimension1=[0 1 2 3 4 5 6 7 8 9 10 11 12 13 14 15 16 17 18 19 20 21 22 23]'  Table=Fncs.Grid_purchase'  ExtrapMethod=Clip  InternalRulePriority=Speed  RndMeth=Simplest
  OUT : Outport
  tag scope: Grd_bit=global, Grid_costs=global
  wires:
  Digital Clock/1 -> MATLAB Function/1(time)
  daily_Grid_costs/1 -> MATLAB Function1/1(u), [Grid_costs]
  MATLAB Function/1(hour_of_day) -> daily_Grid_costs/1
  Subsystem Reference/1 -> To Workspace/1
  [Power_Grid] -> Subsystem Reference/1, OUT/1
  MATLAB Function1/1(y) -> [Grd_bit]

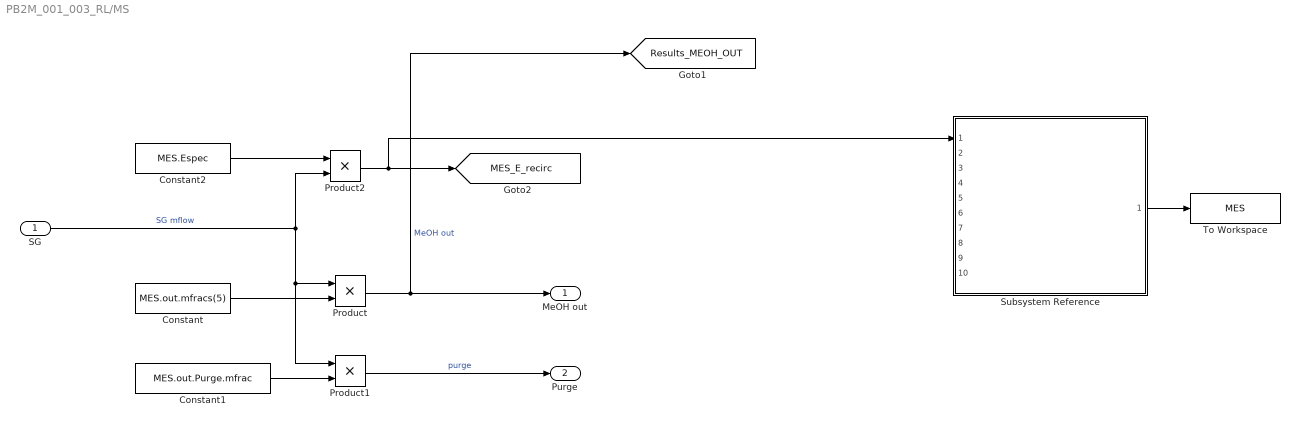
== system PB2M_001_003_RL/MS ==
  SG : Inport
  Constant : Constant  Value=MES.out.mfracs(5)
  Constant1 : Constant  Value=MES.out.Purge.mfrac
  Constant2 : Constant  Value=MES.Espec
  Product : Product
  Product1 : Product
  Product2 : Product
  Subsystem Reference : Subsystem  ReferencedSubsystem=Output_generation
  To Workspace : ToWorkspace  VariableName=MES  SampleTime=-1
  MeOH out : Outport
  Purge : Outport  Port=2
  tag scope: MES_E_recirc=global, Results_MEOH_OUT=global
  wires:
  Subsystem Reference/1 -> To Workspace/1
  Constant/1 -> Product/2
  Constant2/1 -> Product2/1
  Product2/1 -> Subsystem Reference/1, [MES_E_recirc]
  SG/1 -> Product1/1, Product/1, Product2/2  "SG mflow"
  Product/1 -> [Results_MEOH_OUT], MeOH out/1  "MeOH out"
  Product1/1 -> Purge/1  "purge"
  Constant1/1 -> Product1/2

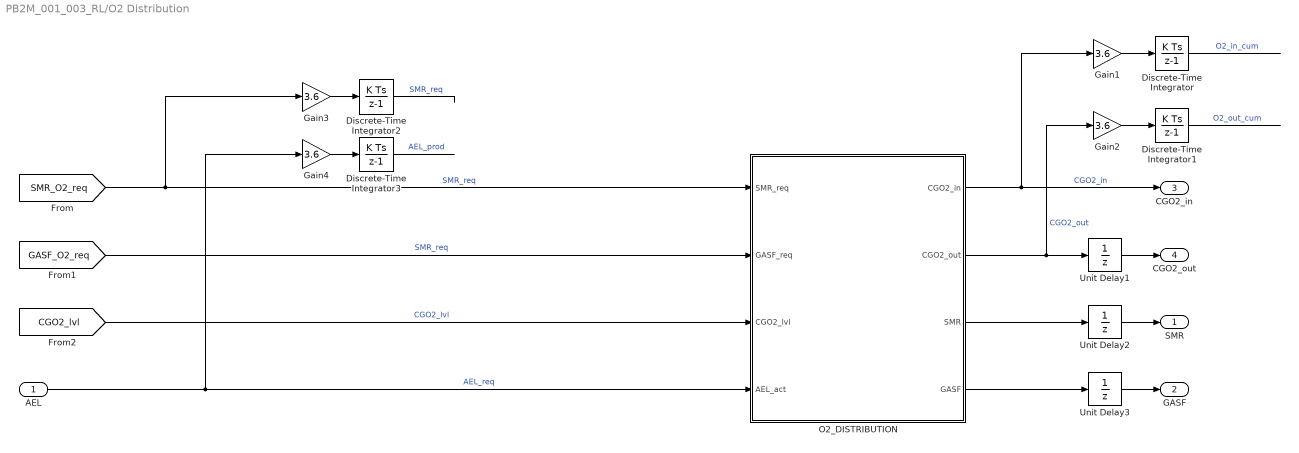
== system PB2M_001_003_RL/O2 Distribution ==
  AEL : Inport
  Discrete-Time Integrator{,1..3} (4 alike) : DiscreteIntegrator  SampleTime=-1  ICPrevOutput=DiscIntNeverNeededParam  ICPrevScaledInput=DiscIntNeverNeededParam
  Gain{1..4} (4 alike) : Gain  Gain=3.6
  O2_DISTRIBUTION : Stateflow chart  TreatAsAtomicUnit=on
      settings: PortSchema="{\"entries\":[{\"content\":{\"sides\":[{\"content\":{\"connectorIds\":[\"In1\",\"In4\",\"In3\",\"In2\"]},\"type\":\"ConnectorPlacement.EquallySpacedRectSide\",\"uuid\":\"621105b3-c3dc-4330-bdef-d993cdecb60c\"},{\"content\":{\"connectorIds\":[\"Out1\",\"Out2\",\"Out3\",\"Out4\"],\"side\":\"RIGHT\"},\"type\":\"ConnectorPlacement.EquallySpacedRectSide\",\"uuid\":\"49dd08d2-12bd-4f9c-8bf9-bd4ad8fb6d9e\"},{\"content\":{\"side\":\"TOP\"},\"type\":\"ConnectorPlacement.EquallySpacedRectSide\",\"uuid\":\"131dd091-cb90-4a7c-ba23-9028845e06c3\"}]},\"type\":\"ConnectorPlacement.EquallySpacedConnector\",\"uuid\":\"78af0694-bd8e-4e4a-a281-7245970286e6\"}],\"packageUris\":[\"http://schema.mathworks.com/mf0/Connector/R2020b\"],\"version\":\"1.0\"}"
  Unit Delay1 : UnitDelay  SampleTime=-1  HasFrameUpgradeWarning=on
  Unit Delay2 : UnitDelay  SampleTime=-1  HasFrameUpgradeWarning=on
  Unit Delay3 : UnitDelay  SampleTime=-1  HasFrameUpgradeWarning=on
  SMR : Outport
  GASF : Outport  Port=2
  CGO2_in : Outport  Port=3
  CGO2_out : Outport  Port=4
  wires:
  [SMR_O2_req] -> O2_DISTRIBUTION/1(SMR_req), Gain3/1  "SMR_req"
  O2_DISTRIBUTION/2(CGO2_out) -> Gain2/1, Unit Delay1/1  "CGO2_out"
  O2_DISTRIBUTION/3(SMR) -> Unit Delay2/1
  O2_DISTRIBUTION/1(CGO2_in) -> Gain1/1, CGO2_in/1  "CGO2_in"
  Unit Delay1/1 -> CGO2_out/1
  [CGO2_lvl] -> O2_DISTRIBUTION/3(CGO2_lvl)  "CGO2_lvl"
  Gain1/1 -> Discrete-Time Integrator/1
  Discrete-Time Integrator/1 -> ?  "O2_in_cum"
  Gain2/1 -> Discrete-Time Integrator1/1
  Discrete-Time Integrator1/1 -> ?  "O2_out_cum"
  Gain3/1 -> Discrete-Time Integrator2/1
  Discrete-Time Integrator2/1 -> ?  "SMR_req"
  Gain4/1 -> Discrete-Time Integrator3/1
  Discrete-Time Integrator3/1 -> ?  "AEL_prod"
  AEL/1 -> Gain4/1, O2_DISTRIBUTION/2(AEL_act)  "AEL_req"
  Unit Delay2/1 -> SMR/1
  Unit Delay3/1 -> GASF/1
  O2_DISTRIBUTION/4(GASF) -> Unit Delay3/1
  [GASF_O2_req] -> O2_DISTRIBUTION/4(GASF_req)  "SMR_req"

== system PB2M_001_003_RL/SG DISTR ==
  Input : Inport
  Minus : Sum  Inputs=+-
  CHP : Outport
  MSR : Outport  Port=2
  tag scope: Results_SG_mflow_2=global, Results_SG_mflow_3=global
  wires:
  [CHP_SG_req] -> [Results_SG_mflow_3], Minus/2, CHP/1
  Input/1 -> Minus/1
  Minus/1 -> [Results_SG_mflow_2], MSR/1

== system PB2M_001_003_RL/SG DISTR1 ==
  Input1 : Inport
  AEL : Inport  Port=2
  Add : Sum
  Output : Outport
  tag scope: Results_SG_mflow_4=global
  wires:
  Input1/1 -> Add/1
  AEL/1 -> Add/2
  Add/1 -> [Results_SG_mflow_4], Output/1

== system PB2M_001_003_RL/WT, PV ==
  Ambient Temperature : Lookup_n-D  NumberOfTableDimensions=1  BreakpointsForDimension1=global_time  Table=[AMB.LU.t_air]'  ExtrapMethod=Clip  InternalRulePriority=Speed  RndMeth=Simplest
  Digital Clock : DigitalClock  SampleTime=[global_ST]
  PHOTOVOLTAIC : Subsystem
  Solar Irradiance : Lookup_n-D  NumberOfTableDimensions=1  BreakpointsForDimension1=global_time  Table=[AMB.LU.G_t]'  ExtrapMethod=Clip  InternalRulePriority=Speed  RndMeth=Simplest
  Sum : Sum
  WIND TURBINE : Subsystem
  Wind Speed : Lookup_n-D  NumberOfTableDimensions=1  BreakpointsForDimension1=global_time  Table=[AMB.LU.v_wind]'  ExtrapMethod=Clip  InternalRulePriority=Speed  RndMeth=Simplest
  P_renew : Outport
  tag scope: Results_P_PV=global, Results_P_WT=global, Results_P_renew=global, T_Amb=global
  wires:
  Solar Irradiance/1 -> PHOTOVOLTAIC/1(G_t [W/m^2])  "G_t"
  Digital Clock/1 -> Wind Speed/1, Ambient Temperature/1, Solar Irradiance/1
  Ambient Temperature/1 -> PHOTOVOLTAIC/2(t_amb [°C]), [T_Amb]  "t_amb"
  Wind Speed/1 -> WIND TURBINE/1(v_wind [m/s])  "v_wind"
  PHOTOVOLTAIC/1(PV_P_Out_MW) -> [Results_P_PV], Sum/1  "P_El_PV"
  Sum/1 -> [Results_P_renew], P_renew/1  "P_El_Total"
  WIND TURBINE/1(WT_P_Out [MW]) -> [Results_P_WT], Sum/2  "P_WT"

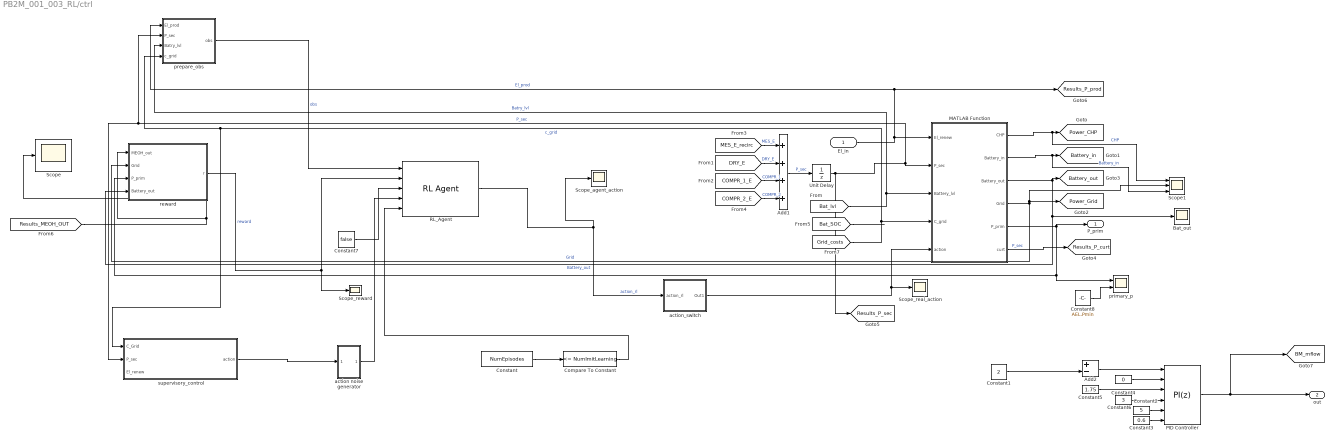
== system PB2M_001_003_RL/ctrl ==
  El_in : Inport
  Add1 : Sum  Inputs=++++
  Add2 : Sum  Inputs=+-
  Bat_out : Scope
  Compare To Constant : simulink/Logic and Bit Operations/Compare To Constant  relop=<=  const=NumImitLearning  OutDataTypeStr=boolean
  Constant : Constant  Value=NumEpisodes
  Constant1 : Constant  Value=2
  Constant2 : Constant  Value=5
  Constant3 : Constant  Value=0.6
  Constant4 : Constant  Value=0
  Constant5 : Constant  Value=1.75
  Constant6 : Constant  Value=3
  Constant7 : Constant  Value=false  SampleTime=1
  Constant8 : Constant  Value=AEL.Pmin
  MATLAB Function : MATLAB Function  TreatAsAtomicUnit=on
  PID Controller : slpidlib/PID Controller  Controller=PI  Form=Parallel  TimeDomain=Discrete-time  UseExternalTs=off  SampleTime=-1  IntegratorMethod=Forward Euler  FilterMethod=Forward Euler  ControllerParametersSource=external  P=0  I=-10  UseKiTs=off  D=0  UseExternalDerivativeSource=off  N=100  UseFilter=on  TunerSelectOption=Transfer Function Based (PID Tuner App)  InitialConditionSource=external  InitialConditionForIntegrator=0.75  InitialConditionForFilter=0  DifferentiatorICPrevScaledInput=0  ExternalReset=none  TrackingMode=off  Kt=1  LimitOutput=on  SatLimitsSource=external  UpperSaturationLimit=1  LowerSaturationLimit=0.5  LinearizeAsGain=on  AntiWindupMode=back-calculation  Kb=1  LimitIntegrator=off  UpperIntegratorSaturationLimit=inf  LowerIntegratorSaturationLimit=-inf  POutMin=[]  POutMax=[]  IOutMin=[]  IOutMax=[]  DOutMin=[]  DOutMax=[]  NOutMin=[]  NOutMax=[]  SumOutMin=[]  SumOutMax=[]  SaturationOutMin=[]  SaturationOutMax=[]  PParamMin=[]  PParamMax=[]  IParamMin=[]  IParamMax=[]  DParamMin=[]  DParamMax=[]  NParamMin=[]  NParamMax=[]  KbParamMin=[]  KbParamMax=[]  KtParamMin=[]  KtParamMax=[]  KbOutMin=[]  KbOutMax=[]  KtOutMin=[]  KtOutMax=[]  IntegratorOutMin=[]  IntegratorOutMax=[]  FilterOutMin=[]  FilterOutMax=[]  SumI1OutMin=[]  SumI1OutMax=[]  SumI2OutMin=[]  SumI2OutMax=[]  SumI3OutMin=[]  SumI3OutMax=[]  SumI4OutMin=[]  SumI4OutMax=[]  SumDOutMin=[]  SumDOutMax=[]  DifferentiatorOutMin=[]  DifferentiatorOutMax=[]  FilterDiffOutCoefMin=[]  FilterDiffOutCoefMax=[]  ReciprocalOutMin=[]  ReciprocalOutMax=[]  SumDenOutMin=[]  SumDenOutMax=[]  SumNumOutMin=[]  SumNumOutMax=[]  DivideOutMin=[]  DivideOutMax=[]  UdiffTsProdOutMin=[]  UdiffTsProdOutMax=[]  NTsProdOutMin=[]  NTsProdOutMax=[]  UintegralTsProdOutMin=[]  UintegralTsProdOutMax=[]  UngainTsProdOutMin=[]  UngainTsProdOutMax=[]  ClampingZeroOutDataTypeStr=Inherit: Inherit via back propagation  ClampingZeroOutMin=[]  ClampingZeroOutMax=[]  FilterDenConstantOutDataTypeStr=Inherit: Inherit via back propagation  FilterDenConstantOutMin=[]  FilterDenConstantOutMax=[]  PCopyOutDataTypeStr=Inherit: Inherit via back propagation  PCopyOutMin=[]  PCopyOutMax=[]  NCopyOutDataTypeStr=Inherit: Inherit via back propagation  NCopyOutMin=[]  NCopyOutMax=[]  IntegratorContinuousStateAttributes=''  IntegratorStateMustResolveToSignalObject=off  IntegratorRTWStateStorageClass=Auto  FilterContinuousStateAttributes=''  FilterStateMustResolveToSignalObject=off  FilterRTWStateStorageClass=Auto  ParallelPVariant=ExternalParameters  IdealPVariant=Disabled  IVariant=ExternalParameters  DVariant=Disabled  IntegratorVariant=Discrete  SatVariant=External  AWVariant=BackCalculation  PCopyVariant=Disabled  TRVariant=Disabled  FdbkBlocksVariant=Forward  IdealPFdbkVariant=Disabled  SatFdbkVariant=Disabled  DerivativeFilterVariant=Disabled  NVariant=Disabled  NCopyVariant=Disabled_SignalSpec  FilterICVariant=Disabled  IntegratorICVariant=ExternalICs  ExternalResetVariant=Disabled  TRSumVariant=Passthrough  SumFdbkVariant=Disabled  SumVariant=Sum_PI  TsampFilterVariant=InternalTs  TsampNgainVariant=Passthrough  TsampIntegralVariant=Disabled_SignalSpec  ExternalSaturationOutDataTypeStr=Inherit: Same as second input  DerivativeSourceVariant=Disabled
  RL_Agent : rllib/RL Agent  Agent=agentObj  ExternalActionAsInput=on  ProvideLastAction=off  ProvideCumRwd=off  TreatAsDirectFeedthrough=on  UseStrictObservationDataTypes=off
  Scope : Scope
  Scope1 : Scope  NumInputPorts=3
  Scope_agent_action : Scope
  Scope_real_action : Scope
  Scope_reward : Scope
  Unit Delay : UnitDelay  SampleTime=-1  HasFrameUpgradeWarning=on
  action noise generator : Subsystem
  action_switch : Subsystem
  prepare_obs : Subsystem
  primary_p : Scope  NumInputPorts=2
  reward : MATLAB Function  TreatAsAtomicUnit=on
  supervisory_control : MATLAB Function  TreatAsAtomicUnit=on
  P_prim : Outport
  out : Outport  Port=2
  tag scope: BM_mflow=global, Battery_in=global, Battery_out=global, Power_CHP=global, Power_Grid=global, Results_P_curt=global, Results_P_prod=global, Results_P_sec=global
  wires:
  [MES_E_recirc] -> Add1/1  "MES_E"
  [Grid_costs] -> prepare_obs/4(c_grid), supervisory_control/1(C_Grid), MATLAB Function/4(C_grid)  "c_grid"
  [DRY_E] -> Add1/2  "DRY_E"
  [COMPR_1_E] -> Add1/3  "COMPR_1"
  [COMPR_2_E] -> Add1/4  "COMPR_2"
  Add1/1 -> Unit Delay/1  "P_sec"
  [Bat_lvl] -> prepare_obs/3(Batry_lvl), MATLAB Function/3(Battery_lvl)  "Batry_lvl"
  El_in/1 -> prepare_obs/1(El_prod), [Results_P_prod], MATLAB Function/1(El_renew)  "El_prod"
  [Bat_SOC] -> ?
  Unit Delay/1 -> [Results_P_sec], supervisory_control/2(P_sec), prepare_obs/2(P_sec), MATLAB Function/2(P_sec)  "P_sec"
  Constant2/1 -> PID Controller/5
  Constant6/1 -> PID Controller/4
  PID Controller/1 -> [BM_mflow], out/1
  Constant1/1 -> Add2/2
  ? -> Add2/1
  Constant5/1 -> PID Controller/3
  Constant4/1 -> PID Controller/2
  Constant3/1 -> PID Controller/6
  Add2/1 -> PID Controller/1
  [Results_MEOH_OUT] -> reward/1(MEOH_out), Scope/1
  MATLAB Function/5(P_prim) -> reward/3(P_prim), primary_p/1, P_prim/1
  reward/1(r) -> RL_Agent/2, Scope_reward/1  "reward"
  MATLAB Function/1(CHP) -> Scope1/1, [Power_CHP]  "CHP"
  MATLAB Function/2(Battery_in) -> Scope1/3, [Battery_in]  "Battery_in"
  MATLAB Function/3(Battery_out) -> reward/4(Battery_out), Bat_out/1, [Battery_out]  "Battery_out"
  MATLAB Function/4(Grid) -> [Power_Grid], Scope1/2, reward/2(Grid)  "Grid"
  MATLAB Function/6(curt) -> [Results_P_curt]  "P_sec"
  RL_Agent/1 -> action_switch/1(action_rl), Scope_agent_action/1  "action_rl"
  action_switch/1(Out1) -> Scope_real_action/1, MATLAB Function/5(action)
  Constant7/1 -> RL_Agent/3
  prepare_obs/1(obs) -> RL_Agent/1  "obs"
  Compare To Constant/1 -> RL_Agent/5
  Constant/1 -> Compare To Constant/1
  supervisory_control/1(action) -> action noise generator/1(action)
  action noise generator/1(Out1) -> RL_Agent/4
  Constant8/1 -> primary_p/2

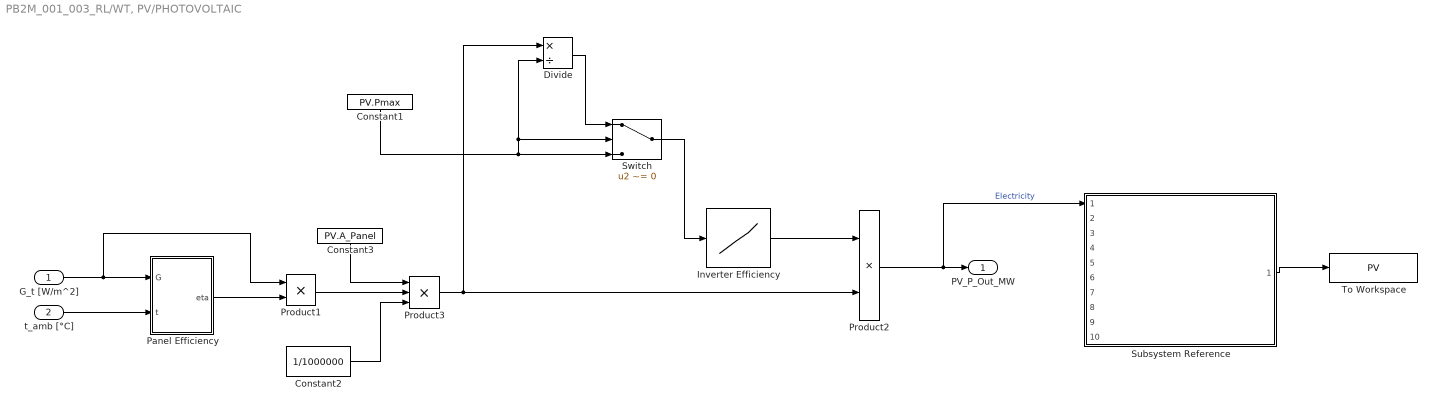
== system PB2M_001_003_RL/WT, PV/PHOTOVOLTAIC ==
  G_t [W/m^2] : Inport
  t_amb [°C] : Inport  Port=2
  Constant1 : Constant  Value=PV.Pmax
  Constant2 : Constant  Value=1/1000000
  Constant3 : Constant  Value=PV.A_Panel
  Divide : Product  Inputs=*/
  Inverter Efficiency : Lookup_n-D  NumberOfTableDimensions=1  BreakpointsForDimension1=[PV.Inv_LU.P_relat]'  Table=[PV.Inv_LU.eta_inv]'  InternalRulePriority=Speed  RndMeth=Simplest
  Panel Efficiency : MATLAB Function  TreatAsAtomicUnit=on
  Product1 : Product
  Product2 : Product
  Product3 : Product  Inputs=3
  Subsystem Reference : Subsystem  ReferencedSubsystem=Output_generation
  Switch : Switch  Criteria=u2 ~= 0  SaturateOnIntegerOverflow=off  InputSameDT=off
  To Workspace : ToWorkspace  VariableName=PV  SampleTime=-1
  PV_P_Out_MW : Outport
  wires:
  G_t [W/m^2]/1 -> Panel Efficiency/1(G), Product1/1
  t_amb [°C]/1 -> Panel Efficiency/2(t)
  Panel Efficiency/1(eta) -> Product1/2
  Product1/1 -> Product3/2
  Inverter Efficiency/1 -> Product2/1
  Product2/1 -> Subsystem Reference/1, PV_P_Out_MW/1  "Electricity"
  Constant3/1 -> Product3/1
  Constant2/1 -> Product3/3
  Product3/1 -> Divide/1, Product2/2
  Divide/1 -> Switch/1
  Switch/1 -> Inverter Efficiency/1
  Constant1/1 -> Divide/2, Switch/2, Switch/3
  Subsystem Reference/1 -> To Workspace/1

== system PB2M_001_003_RL/WT, PV/WIND TURBINE ==
  v_wind [m/s] : Inport
  Add : Sum
  Constant : Constant  Value=WT.n_typeA
  Constant1 : Constant  Value=WT.n_typeB
  Constant2 : Constant  Value=WT.ws_corr_factor
  Product : Product
  Product1 : Product
  Product2 : Product
  Subsystem Reference : Subsystem  ReferencedSubsystem=Output_generation
  To Workspace : ToWorkspace  VariableName=WT  SampleTime=-1
  V112 3.45 MW : Lookup_n-D  NumberOfTableDimensions=1  BreakpointsForDimension1=[WT.PowerCurve.v_wind]'  Table=[WT.PowerCurve.P_WT_3_45]'  InternalRulePriority=Speed  RndMeth=Simplest
  V112 4.2 MW : Lookup_n-D  NumberOfTableDimensions=1  BreakpointsForDimension1=[WT.PowerCurve.v_wind]'  Table=[WT.PowerCurve.P_WT_4_2]'  InternalRulePriority=Speed  RndMeth=Simplest
  WT_P_Out [MW] : Outport
  wires:
  V112 3.45 MW/1 -> Product/2
  Constant/1 -> Product/1
  V112 4.2 MW/1 -> Product1/1
  Constant1/1 -> Product1/2
  Product/1 -> Add/1
  Product1/1 -> Add/2
  Add/1 -> Subsystem Reference/1, WT_P_Out [MW]/1  "Electricity"
  v_wind [m/s]/1 -> Product2/1
  Product2/1 -> V112 3.45 MW/1, V112 4.2 MW/1
  Constant2/1 -> Product2/2
  Subsystem Reference/1 -> To Workspace/1

== system PB2M_001_003_RL/ctrl/action noise generator ==
  action : Inport
  Add : Sum
  Random Number : RandomNumber  Variance=imit_action_noise_variance  Seed=NumEpisodes  SampleTime=1
  Saturation : Saturate  UpperLimit=1  LowerLimit=-1
  Out1 : Outport
  wires:
  Add/1 -> Saturation/1
  Random Number/1 -> Add/2
  action/1 -> Add/1
  Saturation/1 -> Out1/1

== system PB2M_001_003_RL/ctrl/action_switch ==
  action_rl : Inport
  Constant8 : Constant  Value=vanilla  SampleTime=1
  Multiport Switch : MultiPortSwitch  DataPortOrder=Specify indices  DataPortIndices={0,1,2,3}  SaturateOnIntegerOverflow=off  InputSameDT=off
  Switch Case : SwitchCase  CaseConditions={0,1,2,3}  ShowDefaultCase=off
  Switch Case Action Subsystem : Subsystem  TreatAsAtomicUnit=on
  Switch Case Action Subsystem1 : Subsystem  TreatAsAtomicUnit=on
  Switch Case Action Subsystem2 : Subsystem  TreatAsAtomicUnit=on
  Switch Case Action Subsystem3 : Subsystem  TreatAsAtomicUnit=on
  Out1 : Outport
  wires:
  Switch Case Action Subsystem1/1(Out1) -> Multiport Switch/3
  Constant8/1 -> Multiport Switch/1, Switch Case/1
  Switch Case/4 -> Switch Case Action Subsystem3/Action
  Switch Case Action Subsystem/1(action) -> Multiport Switch/2
  Switch Case/3 -> Switch Case Action Subsystem2/Action
  Switch Case/1 -> Switch Case Action Subsystem/Action
  Switch Case/2 -> Switch Case Action Subsystem1/Action
  Switch Case Action Subsystem2/1(Out1) -> Multiport Switch/4
  Switch Case Action Subsystem3/1(Out1) -> Multiport Switch/5
  action_rl/1 -> Switch Case Action Subsystem/1(In1)
  Multiport Switch/1 -> Out1/1

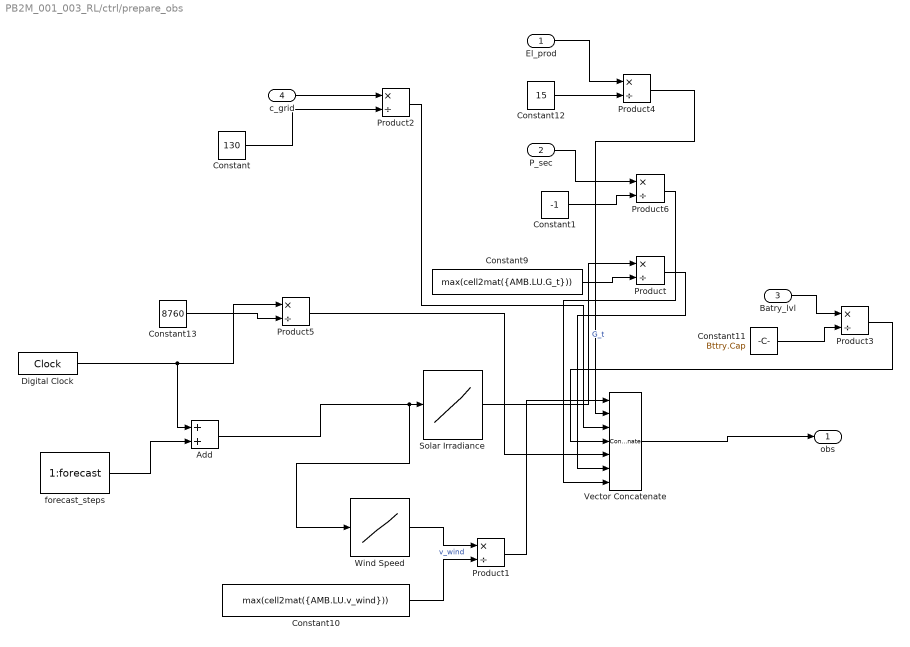
== system PB2M_001_003_RL/ctrl/prepare_obs ==
  El_prod : Inport
  P_sec : Inport  Port=2
  Batry_lvl : Inport  Port=3
  c_grid : Inport  Port=4
  Add : Sum
  Constant : Constant  Value=130
  Constant1 : Constant  Value=-1
  Constant10 : Constant  Value=max(cell2mat({AMB.LU.v_wind}))
  Constant11 : Constant  Value=Bttry.Cap
  Constant12 : Constant  Value=15
  Constant13 : Constant  Value=8760
  Constant9 : Constant  Value=max(cell2mat({AMB.LU.G_t}))
  Digital Clock : DigitalClock
  Product{,1..6} (7 alike) : Product  Inputs=*/
  Solar Irradiance : Lookup_n-D  NumberOfTableDimensions=1  BreakpointsForDimension1=global_time  BreakpointsForDimension2=global_time +2  Table=[AMB.LU.G_t]'  ExtrapMethod=Clip  InternalRulePriority=Speed  RndMeth=Simplest
  Vector Concatenate : Concatenate  NumInputs=7
  Wind Speed : Lookup_n-D  NumberOfTableDimensions=1  BreakpointsForDimension1=global_time  Table=[AMB.LU.v_wind]'  ExtrapMethod=Clip  InternalRulePriority=Speed  RndMeth=Simplest
  forecast_steps : Constant  Value=1:forecast
  obs : Outport
  wires:
  Constant10/1 -> Product1/2
  Product/1 -> Vector Concatenate/6
  Add/1 -> Wind Speed/1, Solar Irradiance/1
  Constant9/1 -> Product/2
  forecast_steps/1 -> Add/2
  Product5/1 -> Vector Concatenate/5
  Product1/1 -> Vector Concatenate/1
  Digital Clock/1 -> Product5/1, Add/1
  Wind Speed/1 -> Product1/1  "v_wind"
  Constant12/1 -> Product4/2
  Solar Irradiance/1 -> Product/1  "G_t"
  Vector Concatenate/1 -> obs/1
  Constant11/1 -> Product3/2
  Product3/1 -> Vector Concatenate/4
  Constant/1 -> Product2/2
  Constant13/1 -> Product5/2
  Batry_lvl/1 -> Product3/1
  El_prod/1 -> Product4/1
  c_grid/1 -> Product2/1
  Product2/1 -> Vector Concatenate/3
  Product4/1 -> Vector Concatenate/2
  Constant1/1 -> Product6/2
  P_sec/1 -> Product6/1
  Product6/1 -> Vector Concatenate/7

== system PB2M_001_003_RL/ctrl/action_switch/Switch Case Action Subsystem ==
  In1 : Inport
  Action Port : ActionPort  ActionPortLabel=case [ 0 ]:
  action : Outport
  wires:
  In1/1 -> action/1

== system PB2M_001_003_RL/ctrl/action_switch/Switch Case Action Subsystem1 ==
  Action Port : ActionPort  ActionPortLabel=case [ 1 ]:
  Constant : Constant  Value=0
  Out1 : Outport
  wires:
  Constant/1 -> Out1/1

== system PB2M_001_003_RL/ctrl/action_switch/Switch Case Action Subsystem2 ==
  Action Port : ActionPort  ActionPortLabel=case [ 2 ]:
  Uniform Random Number : UniformRandomNumber  SampleTime=1
  Out1 : Outport
  wires:
  Uniform Random Number/1 -> Out1/1

== system PB2M_001_003_RL/ctrl/action_switch/Switch Case Action Subsystem3 ==
  Action Port : ActionPort  ActionPortLabel=case [ 3 ]:
  Constant : Constant
  Out1 : Outport
  wires:
  Constant/1 -> Out1/1

== matlab function PB2M_001_003_RL/GRID/MATLAB Function ==
  data: time input; hour_of_day output
function hour_of_day = hour_function(time)

hour_of_day = hour_function_Ex(time);

end

== matlab function PB2M_001_003_RL/ctrl/reward ==
  data: MEOH_out input; Grid input; r output; P_prim input; Battery_out input; AEL parameter
function r = rew(MEOH_out, Grid, P_prim, Battery_out, AEL)
shortage = AEL.Pmin - P_prim - Battery_out - Grid > 0;
if shortage
    r = -(AEL.Pmin - P_prim - Battery_out - Grid)/AEL.Pmin;
 else
     r = 0;%-MEOH_out;
end

== matlab function PB2M_001_003_RL/ctrl/supervisory_control ==
  data: C_Grid input; action output; Grd parameter; P_sec input; El_renew input; AEL parameter

function action = spvsry_ctrl(C_Grid,Grd, P_sec, El_renew, AEL)

    action = 1;
    P_prim = El_renew - P_sec;
    if P_prim < AEL.Pmin
        action = -1;
        if C_Grid <= Grd.cbuy && P_prim < AEL.Pmin
            action = 0;
        end
    end

== stateflow chart PB2M_001_003_RL/O2 Distribution/O2_DISTRIBUTION ==
  state ACTION
    O2_req = SMR_req + GASF_req;
    shortage = O2_req - AEL_act;
    CGO2_maxIn = (CGO2_cap - CGO2_lvl) * 1000 / 720;
    CGO2_maxOut = CGO2_lvl * 1000 / 720;
    state Surplus
      CGO2_out = 0;
      CGO2_in = min(abs(shortage), CGO2_maxIn);
      SMR = SMR_req;
      GASF = GASF_req;
    state Shortage
      CGO2_out = min(shortage, CGO2_maxOut);
      CGO2_in = 0;
      SMR = SMR_req;
      GASF = GASF_req;
    (default) -> Shortage
    Shortage -> Surplus : [shortage <= 0]
    Surplus -> Shortage : [shortage > 0]
  data: SMR_req input; AEL_act input; CGO2_in output; CGO2_out output; SMR output; O2_req local; shortage local; CGO2_lvl input; CGO2_cap constant double =CGO2_cap; CGO2_maxIn local; CGO2_maxOut local; GASF_req input; GASF output

== matlab function PB2M_001_003_RL/WT, PV/PHOTOVOLTAIC/Panel Efficiency ==
  data: G input; eta output; t input; PV parameter
function eta = TotalEff(G, t, PV)

eta = PV_PanelEff_Ex(G, t, PV);

end
